simulink model "simple_HIL"  (R2025a)
settings: Solver=ode8  StartTime=0.0  StopTime=10  FixedStep=0.0001  RelTol=1e-3
settings Model: Creator=jonno  LastModifiedBy=jonno
settings RTWCC: GenCodeOnly=on

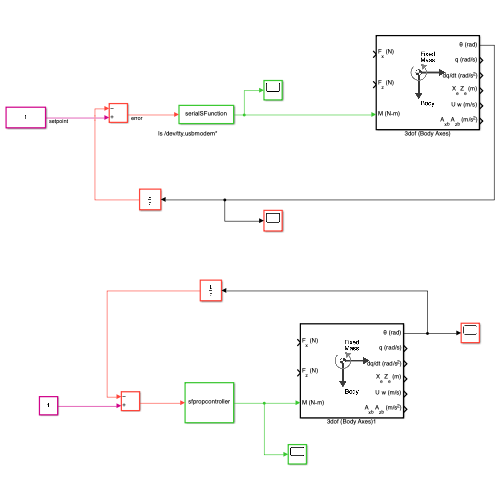
[thumbnail: Simulink's stored preview of the top-level diagram]
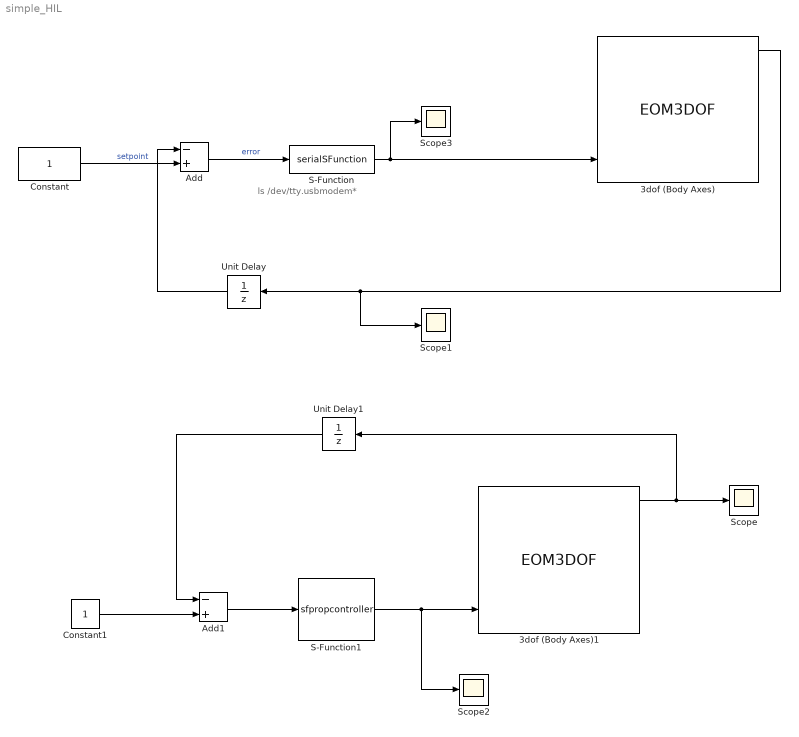
== system simple_HIL ==
  note: ls /dev/tty.usbmodem*
  3dof (Body Axes) : EOM3DOF  v_ini=0  g=0
  3dof (Body Axes)1 : EOM3DOF  v_ini=0  g=0
  Add : Sum  Inputs=-+
  Add1 : Sum  Inputs=-+
  Constant : Constant
  Constant1 : Constant
  S-Function : S-Function  FunctionName=serialSFunction  Parameters='/dev/tty.usbmodem21301'  SFunctionDeploymentMode=off  EnableBusSupport=off
  S-Function1 : S-Function  FunctionName=sfpropcontroller  Parameters=1/100  SFunctionDeploymentMode=off  EnableBusSupport=off
  Scope{,1..3} (4 alike) : Scope
      Scope settings: ActiveDisplayYMinimum=-0.45802289250690831  ActiveDisplayYMaximum=1.8585326242581388
      Scope1 settings: ActiveDisplayYMinimum=0.10516185400632946  ActiveDisplayYMaximum=0.21329404555778719
      Scope2 settings: ActiveDisplayYMinimum=-1.2697055945219229  ActiveDisplayYMaximum=2.4945846245675174  DataLoggingVariableName=ScopeData2
      Scope3 settings: ActiveDisplayYMinimum=18.149324876662089  ActiveDisplayYMaximum=18.673014714976858  DataLoggingVariableName=ScopeData3
  Unit Delay : UnitDelay  SampleTime=-1  HasFrameUpgradeWarning=on
  Unit Delay1 : UnitDelay  SampleTime=-1  HasFrameUpgradeWarning=on
  wires:
  Constant/1 -> Add/2  "setpoint"
  Add/1 -> S-Function/1  "error"
  3dof (Body Axes)/1 -> Scope1/1, Unit Delay/1
  Unit Delay/1 -> Add/1
  3dof (Body Axes)1/1 -> Unit Delay1/1, Scope/1
  Add1/1 -> S-Function1/1
  Constant1/1 -> Add1/2
  S-Function1/1 -> Scope2/1, 3dof (Body Axes)1/3
  Unit Delay1/1 -> Add1/1
  S-Function/1 -> Scope3/1, 3dof (Body Axes)/3
